simulink model "suspension4DOF_2023a"  (R2022b)
settings: Solver=ode5  StartTime=0.0  StopTime=10.0  FixedStep=0.001  RelTol=1e-3
InitFcn:
  | % 悬架参数
  | m_s = 690;
  | I_y = 1222;
  | 
  | lf = 1.25;
  | lr = 1.51;
  | L = lf+lr;
  | 
  | m_uf = 40.5;
  | m_ur = m_uf;
  | 
  | ksf = 17000;
  | ksr = 22000;
  | csf = 1500;
  | csr = 1500;
  | 
  | ktf = 192000;
  | ktr = ktf;
undefined symbols (not defined in the file): road
settings Model: Creator=23649  LastModifiedBy=23649
settings OptimizationCC: ReuseModelBlockBuffer=on
settings RTWCC: GPUComputeCapability=5.0
settings ConfigComp: CovBoundaryAbsTol=1.0e-5

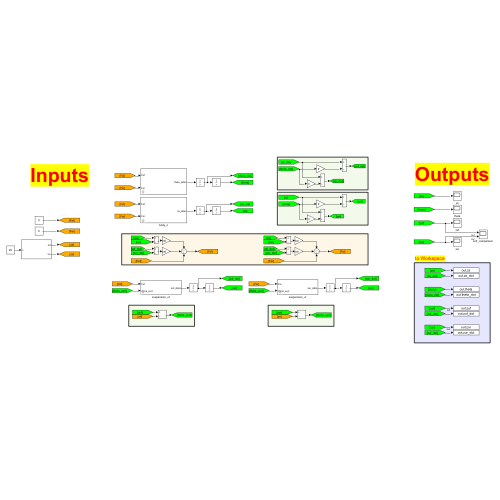
[thumbnail: Simulink's stored preview of the top-level diagram]
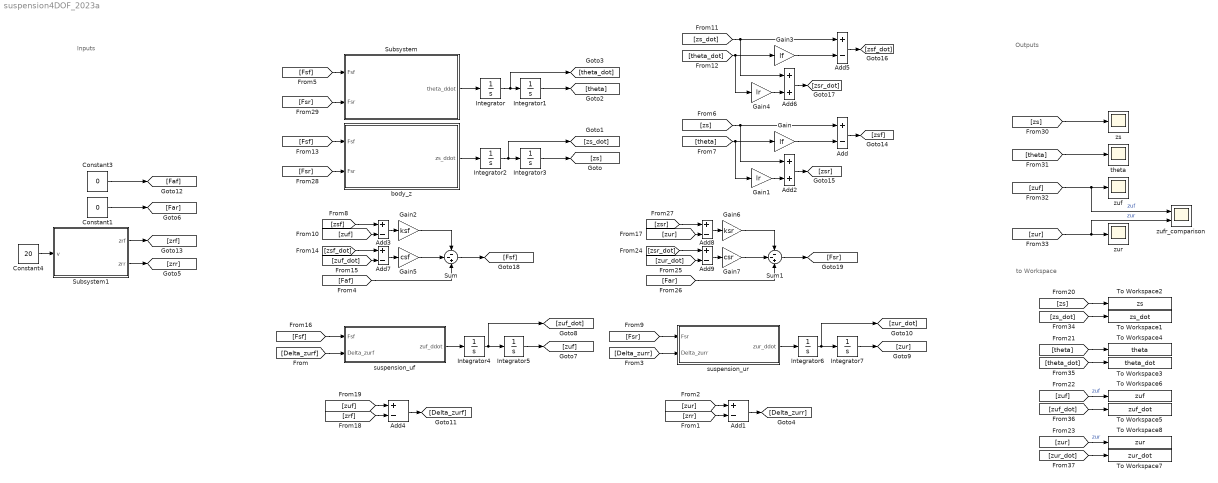
== system suspension4DOF_2023a ==
  note: Inputs
  note: Outputs
  note: to Workspace
  Add{,1,3..5,7..9} (8 alike) : Sum  Inputs=+-
  Add2 : Sum
  Add6 : Sum
  Constant1 : Constant  Value=0
  Constant3 : Constant  Value=0
  Constant4 : Constant  Value=20
  Gain : Gain  Gain=lf
  Gain1 : Gain  Gain=lr
  Gain2 : Gain  Gain=ksf
  Gain3 : Gain  Gain=lf
  Gain4 : Gain  Gain=lr
  Gain5 : Gain  Gain=csf
  Gain6 : Gain  Gain=ksr
  Gain7 : Gain  Gain=csr
  Integrator{,1..7} (8 alike) : Integrator
  Subsystem : Subsystem
      mask DialogControl ParameterGroupVar Prompt: 参数
  Subsystem1 : Subsystem
  Sum : Sum  Inputs=--+
  Sum1 : Sum  Inputs=--+
  To Workspace1 : ToWorkspace  VariableName=zs_dot  SampleTime=-1
  To Workspace2 : ToWorkspace  VariableName=zs  SampleTime=-1
  To Workspace3 : ToWorkspace  VariableName=theta_dot  SampleTime=-1
  To Workspace4 : ToWorkspace  VariableName=theta  SampleTime=-1
  To Workspace5 : ToWorkspace  VariableName=zuf_dot  SampleTime=-1
  To Workspace6 : ToWorkspace  VariableName=zuf  SampleTime=-1
  To Workspace7 : ToWorkspace  VariableName=zur_dot  SampleTime=-1
  To Workspace8 : ToWorkspace  VariableName=zur  SampleTime=-1
  body_z : Subsystem
      mask DialogControl ParameterGroupVar Prompt: 参数
  suspension_uf : Subsystem
      mask DialogControl ParameterGroupVar Prompt: 参数
  suspension_ur : Subsystem
      mask DialogControl ParameterGroupVar Prompt: 参数
  theta : Scope
  zs : Scope
  zuf : Scope
  zufr_comparison : Scope  NumInputPorts=2
  zur : Scope
  wires:
  Constant3/1 -> [Faf]
  Subsystem/1(theta_ddot) -> Integrator/1
  Integrator/1 -> [theta_dot], Integrator1/1
  Integrator2/1 -> [zs_dot], Integrator3/1
  body_z/1(zs_ddot) -> Integrator2/1
  Integrator3/1 -> [zs]
  Integrator1/1 -> [theta]
  Add4/1 -> [Delta_zurf]
  [zuf] -> Add4/1
  [zrf] -> Add4/2
  [zur] -> Add1/1
  Add1/1 -> [Delta_zurr]
  [zrr] -> Add1/2
  Constant1/1 -> [Far]
  [Delta_zurf] -> suspension_uf/2(Delta_zurf)
  [Delta_zurr] -> suspension_ur/2(Delta_zurr)
  Integrator5/1 -> [zuf]
  Integrator4/1 -> [zuf_dot], Integrator5/1
  suspension_uf/1(zuf_ddot) -> Integrator4/1
  Integrator6/1 -> Integrator7/1, [zur_dot]
  Integrator7/1 -> [zur]
  suspension_ur/1(zur_ddot) -> Integrator6/1
  Add/1 -> [zsf]
  [zs] -> Add/1, Add2/1
  [theta] -> Gain1/1, Gain/1
  Gain/1 -> Add/2
  Add2/1 -> [zsr]
  Gain1/1 -> Add2/2
  [zuf] -> Add3/2
  [zsf] -> Add3/1
  Add3/1 -> Gain2/1
  Gain2/1 -> Sum/1
  Gain4/1 -> Add6/2
  Add6/1 -> [zsr_dot]
  Gain3/1 -> Add5/2
  [theta_dot] -> Gain3/1, Gain4/1
  [zs_dot] -> Add6/1, Add5/1
  Add5/1 -> [zsf_dot]
  Add7/1 -> Gain5/1
  [zsf_dot] -> Add7/1
  [zuf_dot] -> Add7/2
  Gain5/1 -> Sum/2
  [Faf] -> Sum/3
  Sum/1 -> [Fsf]
  [Fsf] -> suspension_uf/1(Fsf)
  Sum1/1 -> [Fsr]
  [Far] -> Sum1/3
  Gain7/1 -> Sum1/2
  [zur_dot] -> Add9/2
  [zsr_dot] -> Add9/1
  Add9/1 -> Gain7/1
  Gain6/1 -> Sum1/1
  Add8/1 -> Gain6/1
  [zsr] -> Add8/1
  [zur] -> Add8/2
  [Fsr] -> suspension_ur/1(Fsr)
  [Fsr] -> body_z/2(Fsr)
  [Fsf] -> body_z/1(Fsf)
  [Fsf] -> Subsystem/1(Fsf)
  [Fsr] -> Subsystem/2(Fsr)
  [zs] -> zs/1
  [theta] -> theta/1
  [zuf] -> zufr_comparison/1, zuf/1  "zuf"
  [zur] -> zufr_comparison/2, zur/1  "zur"
  Constant4/1 -> Subsystem1/1(v)
  Subsystem1/2(zrr) -> [zrr]
  Subsystem1/1(zrf) -> [zrf]
  [zs] -> To Workspace2/1
  [zs_dot] -> To Workspace1/1
  [theta] -> To Workspace4/1
  [theta_dot] -> To Workspace3/1
  [zuf] -> To Workspace6/1  "zuf"
  [zuf_dot] -> To Workspace5/1
  [zur] -> To Workspace8/1  "zur"
  [zur_dot] -> To Workspace7/1

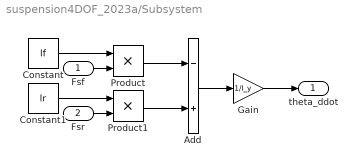
== system suspension4DOF_2023a/Subsystem ==
  Fsf : Inport
  Fsr : Inport  Port=2
  Add : Sum  Inputs=-+
  Constant : Constant  Value=lf
  Constant1 : Constant  Value=lr
  Gain : Gain  Gain=1/I_y
  Product : Product
  Product1 : Product
  theta_ddot : Outport
  wires:
  Fsr/1 -> Product1/2
  Product/1 -> Add/1
  Constant/1 -> Product/1
  Constant1/1 -> Product1/1
  Add/1 -> Gain/1
  Fsf/1 -> Product/2
  Product1/1 -> Add/2
  Gain/1 -> theta_ddot/1

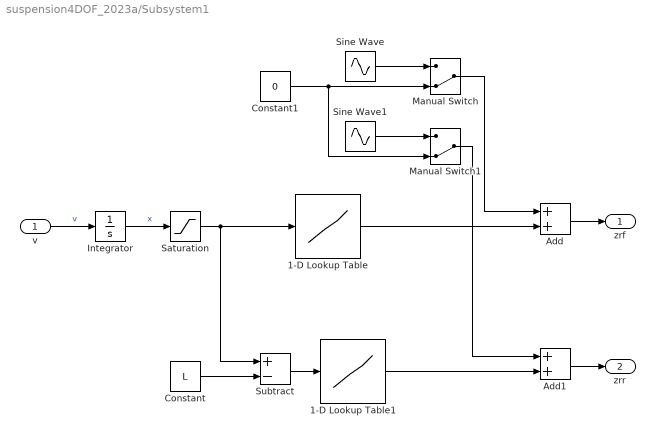
== system suspension4DOF_2023a/Subsystem1 ==
  v : Inport
  1-D Lookup Table : Lookup_n-D  NumberOfTableDimensions=1  BreakpointsForDimension1=road.x  Table=road.z  ExtrapMethod=Clip  InternalRulePriority=Speed  RndMeth=Simplest
  1-D Lookup Table1 : Lookup_n-D  NumberOfTableDimensions=1  BreakpointsForDimension1=road.x  Table=road.z  ExtrapMethod=Clip  InternalRulePriority=Speed  RndMeth=Simplest
  Add : Sum
  Add1 : Sum
  Constant : Constant  Value=L
  Constant1 : Constant  Value=0
  Integrator : Integrator
  Manual Switch : ManualSwitch  CurrentSetting=0
  Manual Switch1 : ManualSwitch  CurrentSetting=0
  Saturation : Saturate  UpperLimit=road.L-road.dx  LowerLimit=0
  Sine Wave : Sin  Amplitude=0.1  Frequency=5  SampleTime=0
  Sine Wave1 : Sin  Amplitude=0.1  Frequency=5  Phase=12  SampleTime=0
  Subtract : Sum  Inputs=+-
  zrf : Outport
  zrr : Outport  Port=2
  wires:
  v/1 -> Integrator/1  "v"
  Integrator/1 -> Saturation/1  "x"
  Saturation/1 -> Subtract/1, 1-D Lookup Table/1
  Subtract/1 -> 1-D Lookup Table1/1
  Constant/1 -> Subtract/2
  Manual Switch/1 -> Add/1
  Manual Switch1/1 -> Add1/1
  Add/1 -> zrf/1
  Add1/1 -> zrr/1
  1-D Lookup Table1/1 -> Add1/2
  1-D Lookup Table/1 -> Add/2
  Sine Wave1/1 -> Manual Switch1/1
  Sine Wave/1 -> Manual Switch/1
  Constant1/1 -> Manual Switch1/2, Manual Switch/2

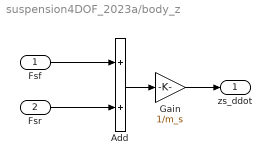
== system suspension4DOF_2023a/body_z ==
  Fsf : Inport
  Fsr : Inport  Port=2
  Add : Sum
  Gain : Gain  Gain=1/m_s
  zs_ddot : Outport
  wires:
  Add/1 -> Gain/1
  Fsf/1 -> Add/1
  Fsr/1 -> Add/2
  Gain/1 -> zs_ddot/1

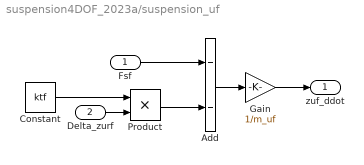
== system suspension4DOF_2023a/suspension_uf ==
  Fsf : Inport
  Delta_zurf : Inport  Port=2
  Add : Sum  Inputs=--
  Constant : Constant  Value=ktf
  Gain : Gain  Gain=1/m_uf
  Product : Product
  zuf_ddot : Outport
  wires:
  Gain/1 -> zuf_ddot/1
  Fsf/1 -> Add/1
  Add/1 -> Gain/1
  Product/1 -> Add/2
  Delta_zurf/1 -> Product/2
  Constant/1 -> Product/1

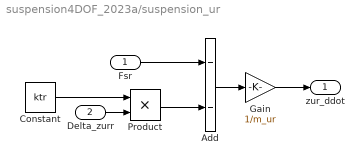
== system suspension4DOF_2023a/suspension_ur ==
  Fsr : Inport
  Delta_zurr : Inport  Port=2
  Add : Sum  Inputs=--
  Constant : Constant  Value=ktr
  Gain : Gain  Gain=1/m_ur
  Product : Product
  zur_ddot : Outport
  wires:
  Constant/1 -> Product/1
  Delta_zurr/1 -> Product/2
  Product/1 -> Add/2
  Add/1 -> Gain/1
  Fsr/1 -> Add/1
  Gain/1 -> zur_ddot/1
